simulink model "boat_dynamics_model"  (R2025a)
settings: Solver=ode4  StartTime=0.0  StopTime=10.0  FixedStep=1e-3  RelTol=1e-3
libraries: simulink_extras x3
settings Model: Creator=brzan  LastModifiedBy=brzan

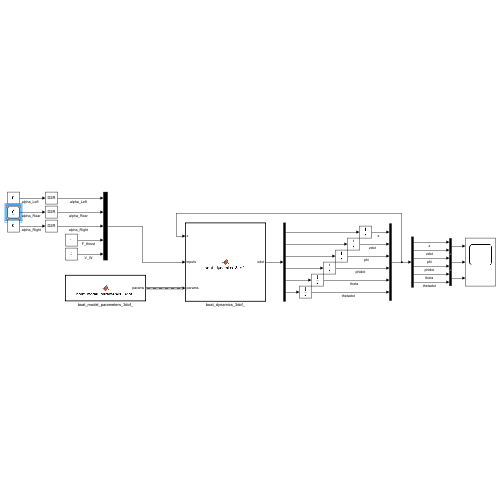
[thumbnail: Simulink's stored preview of the top-level diagram]
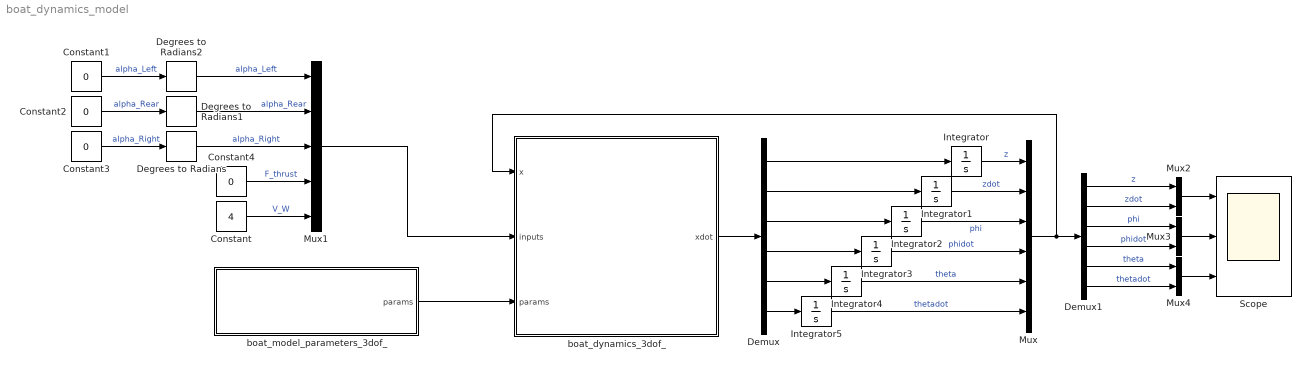
== system boat_dynamics_model ==
  Constant : Constant  Value=4
  Constant{1..4} (4 alike) : Constant  Value=0
  Degrees to Radians : simulink_extras/Transformations/Degrees to Radians
  Degrees to Radians1 : simulink_extras/Transformations/Degrees to Radians
  Degrees to Radians2 : simulink_extras/Transformations/Degrees to Radians
  Demux : Demux  Outputs=6
  Demux1 : Demux  Outputs=6
  Integrator{,1..5} (6 alike) : Integrator
  Mux : Mux  Inputs=6
  Mux1 : Mux  Inputs=5
  Mux2 : Mux  Inputs=2
  Mux3 : Mux  Inputs=2
  Mux4 : Mux  Inputs=2
  Scope : Scope  NumInputPorts=3
      settings: ActiveDisplayYMinimum=-8.05902147455223  ActiveDisplayYMaximum=72.531193270970078
  boat_dynamics_3dof_ : MATLAB Function  TreatAsAtomicUnit=on
  boat_model_parameters_3dof_ : MATLAB Function  TreatAsAtomicUnit=on
  wires:
  boat_dynamics_3dof_/1(xdot) -> Demux/1
  Mux/1 -> Demux1/1, boat_dynamics_3dof_/1(x)
  boat_model_parameters_3dof_/1(params) -> boat_dynamics_3dof_/3(params)
  Demux/1 -> Integrator/1
  Demux/2 -> Integrator1/1
  Demux/4 -> Integrator3/1
  Demux/3 -> Integrator2/1
  Demux/5 -> Integrator4/1
  Demux/6 -> Integrator5/1
  Integrator/1 -> Mux/1  "z"
  Integrator1/1 -> Mux/2  "zdot"
  Integrator2/1 -> Mux/3  "phi"
  Integrator3/1 -> Mux/4  "phidot"
  Integrator4/1 -> Mux/5  "theta"
  Integrator5/1 -> Mux/6  "thetadot"
  Constant/1 -> Mux1/5  "V_W"
  Degrees to Radians2/1 -> Mux1/1  "alpha_Left"
  Degrees to Radians1/1 -> Mux1/2  "alpha_Rear"
  Constant4/1 -> Mux1/4  "F_thrust"
  Degrees to Radians/1 -> Mux1/3  "alpha_Right"
  Mux1/1 -> boat_dynamics_3dof_/2(inputs)
  Demux1/1 -> Mux2/1  "z"
  Mux2/1 -> Scope/1
  Demux1/2 -> Mux2/2  "zdot"
  Demux1/4 -> Mux3/2  "phidot"
  Demux1/3 -> Mux3/1  "phi"
  Demux1/6 -> Mux4/2  "thetadot"
  Demux1/5 -> Mux4/1  "theta"
  Mux3/1 -> Scope/2
  Mux4/1 -> Scope/3
  Constant3/1 -> Degrees to Radians/1  "alpha_Right"
  Constant2/1 -> Degrees to Radians1/1  "alpha_Rear"
  Constant1/1 -> Degrees to Radians2/1  "alpha_Left"

== matlab function boat_dynamics_model/boat_dynamics_3dof_ ==
  data: x input; xdot output; inputs input; params input Bus: boat_model_parameters size=1
function xdot = boat_dynamics_3dof_(x, inputs, params)
%#codegen
    xdot = boat_dynamics_3dof(x, inputs, params);
end

== matlab function boat_dynamics_model/boat_model_parameters_3dof_ ==
  data: params output Bus: boat_model_parameters size=1
function params = boat_model_parameters_3dof_()
    params = boat_model_parameters_3dof();
end
